simulink model "Lab"  (R2016a)
settings: Solver=VariableStepAuto  StartTime=0.0  StopTime=10.0  RelTol=1e-3
libraries: dspsrcs4 x1
settings Model: Creator=DELL  LastModifiedBy=DELL

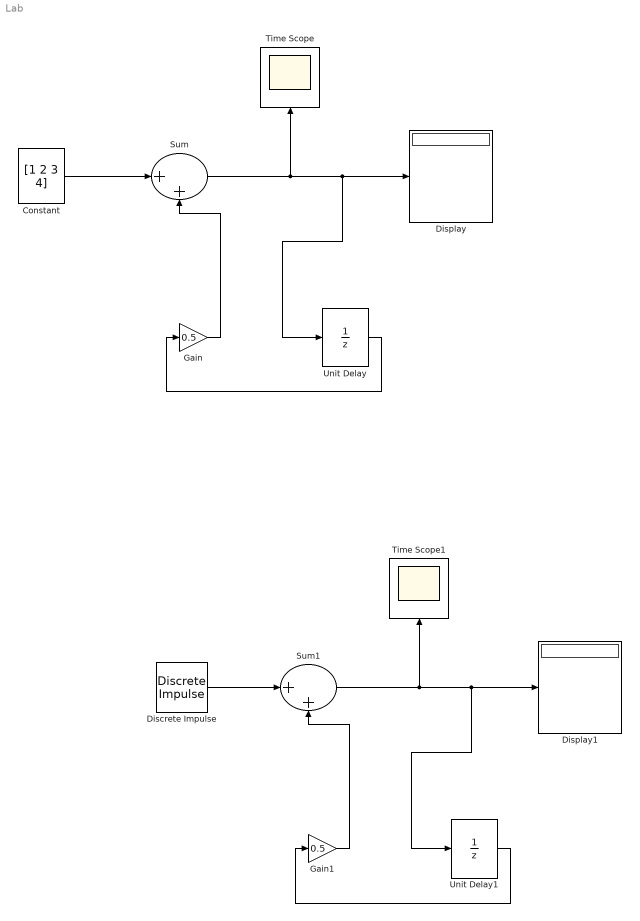
== system Lab ==
  Constant : Constant  Value=[1 2 3 4]  SampleTime=1e-1
  Discrete Impulse : dspsrcs4/Discrete  Impulse  Delay=3  SampleTime=1  FrameSample=1  OutputFrames=off  dataType=double  isSigned=on  wordLen=16  udDataType=sfix(16)  fracBitsMode=Best precision  numFracBits=15  OutDataTypeStr=double  LastOutDataTypeStr=double
  Display : Display
  Display1 : Display
  Gain : Gain  Gain=0.5
  Gain1 : Gain  Gain=0.5
  Sum : Sum  Inputs=|++
  Sum1 : Sum  Inputs=|++
  Time Scope : Scope
  Time Scope1 : Scope
  Unit Delay : UnitDelay  SampleTime=-1
  Unit Delay1 : UnitDelay  SampleTime=-1
  wires:
  Constant/1 -> Sum/1
  Sum/1 -> Time Scope/1, Unit Delay/1, Display/1
  Gain/1 -> Sum/2
  Unit Delay/1 -> Gain/1
  Discrete Impulse/1 -> Sum1/1
  Sum1/1 -> Time Scope1/1, Unit Delay1/1, Display1/1
  Gain1/1 -> Sum1/2
  Unit Delay1/1 -> Gain1/1
